simulink model "smash_exp"  (R2016a)
settings: Solver=VariableStepAuto  StartTime=0.0  StopTime=100  RelTol=1e-3
values from neighbouring files (symbols this model uses):
  in =     [uav_config.mat]
  o =     [uav_config.mat]
libraries: aerolibasang x3, aerolib3dof2 x1, aerolibatmos2 x1, aerolibadyn x1
settings Model: Creator=Bilal  LastModifiedBy=Bilal

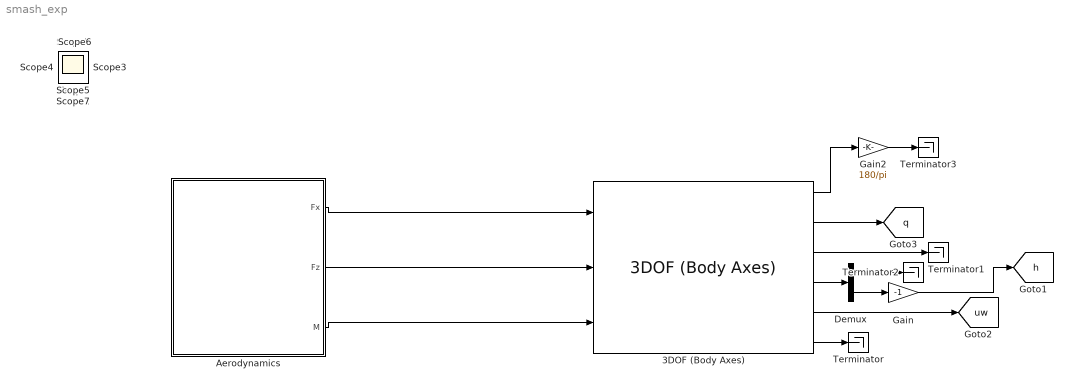
== system smash_exp ==
  3DOF (Body Axes) : aerolib3dof2/3DOF (Body Axes)  units=English (Velocity in kts)  mtype=Fixed  v_ini=in.v.cr  theta_ini=0*pi/180  alpha_ini=0*pi/180  q_ini=0  pos_ini=[0 -in.alt.cr]  mass=o.w0/32.2  mass_e=0.5  mass_f=3.0  Iyy=o.Iyy  Iyy_e=0.5  Iyy_f=3.0  g_in=Internal  g=32.2  vre_flag=on
  Aerodynamics : Subsystem
  Demux : Demux  Outputs=2
  Gain : Gain  Gain=-1
  Gain2 : Gain  Gain=180/pi
  Terminator{,1..3} (4 alike) : Terminator
  Scope{,1..7} (8 alike) : Scope
  tag scope: h=global, q=global, uw=global
  wires:
  3DOF (Body Axes)/4 -> Demux/1
  Demux/2 -> Gain/1
  3DOF (Body Axes)/6 -> Terminator/1
  Gain/1 -> [h]
  Aerodynamics/1(Fx) -> 3DOF (Body Axes)/1
  Aerodynamics/2(Fz) -> 3DOF (Body Axes)/2
  Aerodynamics/3(M) -> 3DOF (Body Axes)/3
  3DOF (Body Axes)/2 -> [q]
  3DOF (Body Axes)/3 -> Terminator1/1
  Demux/1 -> Terminator2/1
  3DOF (Body Axes)/5 -> [uw]
  3DOF (Body Axes)/1 -> Gain2/1
  Gain2/1 -> Terminator3/1

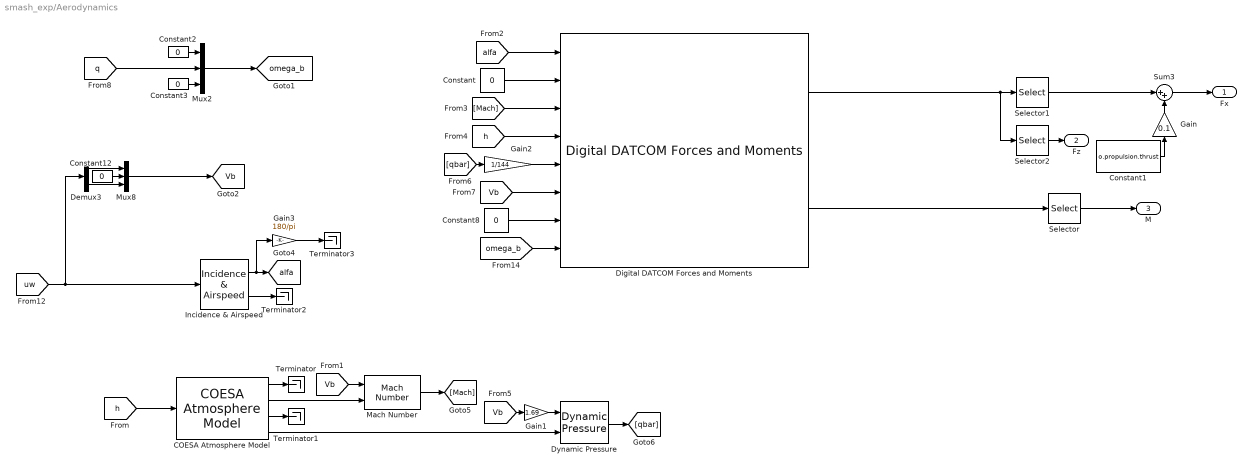
== system smash_exp/Aerodynamics ==
  COESA Atmosphere Model : aerolibatmos2/COESA Atmosphere Model  units=English (Velocity in kts)  spec=1976 COESA-extended U.S. Standard Atmosphere  model=Profile  profile_var=High temperature  profile_percent=1%  profile_alt=5 km (16404 ft)  envelope_var=High temperature  envelope_percent=1%  action=Warning
  Constant{,2..3,8,12} (5 alike) : Constant  Value=0
  Constant1 : Constant  Value=o.propulsion.thrust
  Demux3 : Demux  Outputs=2
  Digital DATCOM Forces and Moments : aerolibadyn/Digital DATCOM Forces and Moments  units=English (Velocity in kts)  dcase=o.aero_dc{1}  fmode=Body  buildno=0  imethod=None - flat  emethod=None - clip  rmethod=Clip to Range  action=None
  Dynamic Pressure : aerolibasang/Dynamic Pressure
  Gain : Gain  Gain=0.1
  Gain1 : Gain  Gain=1.69
  Gain2 : Gain  Gain=1/144
  Gain3 : Gain  Gain=180/pi
  Incidence & Airspeed : aerolibasang/Incidence  & Airspeed
  Mach Number : aerolibasang/Mach Number
  Mux2 : Mux  Inputs=3
  Mux8 : Mux  Inputs=3
  Selector : Selector  InputPortWidth=3  IndexOptions=Index vector (dialog)  Indices=2  OutputSizes=1
  Selector1 : Selector  InputPortWidth=3  IndexOptions=Index vector (dialog)  Indices=1  OutputSizes=1
  Selector2 : Selector  InputPortWidth=3  IndexOptions=Index vector (dialog)  Indices=3  OutputSizes=1
  Sum3 : Sum  Inputs=|++
  Terminator{,1..3} (4 alike) : Terminator
  Fx : Outport  Unit=N
  Fz : Outport  Port=2  Unit=N
  M : Outport  Port=3  Unit=N*m
  tag scope: Vb=global, alfa=global, omega_b=global
  wires:
  Constant/1 -> Digital DATCOM Forces and Moments/2
  [h] -> COESA Atmosphere Model/1
  [Vb] -> Mach Number/1
  COESA Atmosphere Model/1 -> Terminator/1
  COESA Atmosphere Model/3 -> Terminator1/1
  Mach Number/1 -> [Mach]
  [h] -> Digital DATCOM Forces and Moments/4
  [alfa] -> Digital DATCOM Forces and Moments/1
  COESA Atmosphere Model/4 -> Dynamic Pressure/2
  Dynamic Pressure/1 -> [qbar]
  [Vb] -> Digital DATCOM Forces and Moments/6
  Constant8/1 -> Digital DATCOM Forces and Moments/7
  Digital DATCOM Forces and Moments/2 -> Selector/1
  Selector/1 -> M/1
  Selector2/1 -> Fz/1
  Digital DATCOM Forces and Moments/1 -> Selector2/1, Selector1/1
  Incidence & Airspeed/1 -> Gain3/1, [alfa]
  Incidence & Airspeed/2 -> Terminator2/1
  COESA Atmosphere Model/2 -> Mach Number/2
  Demux3/2 -> Mux8/3
  Constant12/1 -> Mux8/2
  Demux3/1 -> Mux8/1
  [uw] -> Incidence & Airspeed/1, Demux3/1
  Mux8/1 -> [Vb]
  Selector1/1 -> Sum3/1
  Sum3/1 -> Fx/1
  Constant1/1 -> Gain/1
  Gain/1 -> Sum3/2
  [q] -> Mux2/2
  Constant2/1 -> Mux2/1
  Constant3/1 -> Mux2/3
  Mux2/1 -> [omega_b]
  [omega_b] -> Digital DATCOM Forces and Moments/8
  [Mach] -> Digital DATCOM Forces and Moments/3
  [Vb] -> Gain1/1
  Gain1/1 -> Dynamic Pressure/1
  [qbar] -> Gain2/1
  Gain2/1 -> Digital DATCOM Forces and Moments/5
  Gain3/1 -> Terminator3/1
